simulink model "Examen_Sim3_v1"  (R2022a)
settings: Solver=VariableStepAuto  StartTime=0.0  StopTime=10  RelTol=1e-3
values from neighbouring files (symbols this model uses):
  A = [22 7 11;-64 -19 -26;-26 -8 -16]    [untitled2.m]
  B = [2;-4;-3]    [untitled2.m]
undefined symbols (not defined in the file or in its folder): C, D, K1, x0
settings Model: Creator=fernando  LastModifiedBy=fernando

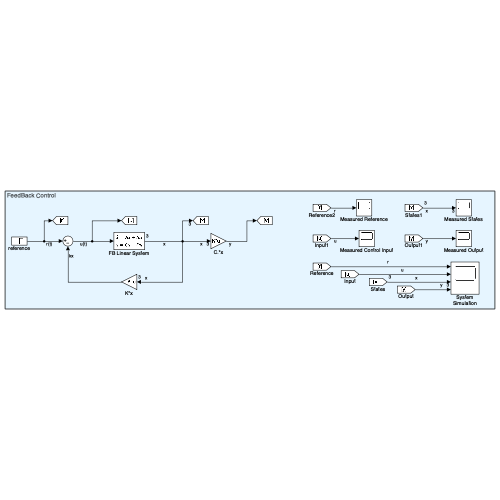
[thumbnail: Simulink's stored preview of the top-level diagram]
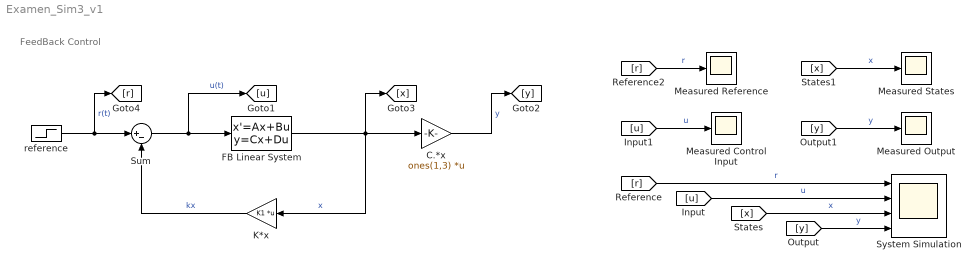
== system Examen_Sim3_v1 ==
  note: FeedBack Control
  C.*x : Gain  Gain=ones(1,3)  Multiplication=Matrix(K*u)
  FB Linear System : StateSpace  A=A  B=B  C=C  D=D  InitialCondition=x0
  K*x : Gain  Gain=K1  Multiplication=Matrix(K*u)
  Measured Control Input : Scope
  Measured Output : Scope
  Measured Reference : Scope
  Measured States : Scope
  Sum : Sum  Inputs=|+-
  System Simulation : Scope  NumInputPorts=4
  reference : Step  SampleTime=0
  wires:
  FB Linear System/1 -> [x], K*x/1, C.*x/1  "x"
  C.*x/1 -> [y]  "y"
  K*x/1 -> Sum/2  "kx"
  Sum/1 -> FB Linear System/1, [u]  "u(t)"
  [r] -> System Simulation/1  "r"
  [u] -> System Simulation/2  "u"
  [x] -> System Simulation/3  "x"
  [y] -> System Simulation/4  "y"
  [r] -> Measured Reference/1  "r"
  [x] -> Measured States/1  "x"
  [y] -> Measured Output/1  "y"
  [u] -> Measured Control Input/1  "u"
  reference/1 -> [r], Sum/1  "r(t)"
